simulink model "rectifysinglephase"  (Simulink 7.8)
settings: Solver=ode45  StartTime=0.0  StopTime=0.1  RelTol=1e-3
libraries: powerlib x9
settings Model: Creator=Administrator  LastModifiedBy=赵
settings DebuggingCC: FcnCallInpInsideContextMsg=Use local settings  StrictBusMsg=Warning

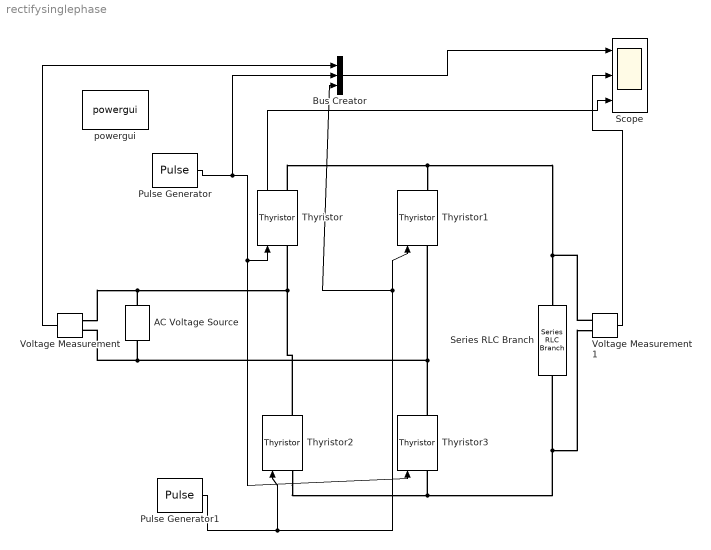
== system rectifysinglephase ==
  AC Voltage Source : powerlib/Electrical Sources/AC Voltage Source  Amplitude=100  Phase=0  Frequency=50  SampleTime=0  Measurements=None
  Bus Creator : BusCreator  Inputs=3
  Pulse Generator : DiscretePulseGenerator  PulseType=Time based  Amplitude=10  Period=0.02  PulseWidth=10  PhaseDelay=60/360*0.02
  Pulse Generator1 : DiscretePulseGenerator  PulseType=Time based  Amplitude=10  Period=0.02  PulseWidth=10  PhaseDelay=(60+180)/360*0.02
  Scope : Scope  NumInputPorts=3
      settings: YMin=-5~-5~-5  YMax=5~5~5
  Series RLC Branch : powerlib/Elements/Series RLC Branch  LConnTagsString=__new0  RConnTagsString=__new0  BranchType=RL  Resistance=2  Inductance=1  SetiL0=off  InitialCurrent=0  Capacitance=1e-6  Setx0=off  InitialVoltage=0  Measurements=None
  Thyristor{,1..3} (4 alike) : powerlib/Power Electronics/Thyristor  Ron=0.001  Lon=0  Vf=0.8  IC=0  Rs=500  Cs=250e-9  Measurements=on
  Voltage Measurement : powerlib/Measurements/Voltage Measurement  PhasorSimulation=off  OutputType=Complex  PSBequivalent=0
  Voltage Measurement1 : powerlib/Measurements/Voltage Measurement  PhasorSimulation=off  OutputType=Complex  PSBequivalent=0
  powergui : powerlib/powergui  Priority=1  SimulationMode=Continuous  SolverType=Tustin  SampleTime=50e-6  frequency=60  SPID=off  DisableSnubberDevices=off  DisableRonSwitches=off  DisableVfSwitches=off  SwTol=0  Interpol=off  DisplayEquations=off  FunctionMessages=off  frequencyindice=50  Pbase=100e6  ErrMax=1e-4  Iterations=50  UnitsV=kV  UnitsW=MW  echomessages=off  HookPort=off  EnableUseOfTLC=off  x0status=blocks  RestoreLinks=warning  ResistiveCurrentMeasurement=off  Frange=[0:2:500]  Ylog=off  Xlog=on  ShowGrid=off  save=off  variable=ZData  ZoomFFT=on  StartTime=0.0  cycles=1  DisplayStyle=1  fundamental=60  FreqAxis=off  MaxFrequency=1000  frequencyindicesteady=1  RmsSteady=1  display=off  Ts=0  methode=off
  wires:
  Pulse Generator/1 -> Thyristor/1, Thyristor3/1, Bus Creator/2
  Pulse Generator1/1 -> Thyristor2/1, Thyristor1/1, Bus Creator/3
  Voltage Measurement/1 -> Bus Creator/1
  Bus Creator/1 -> Scope/1
  Thyristor/1 -> Scope/3
  Voltage Measurement1/1 -> Scope/2
  connections:
  Voltage Measurement/LConn1 -- Thyristor2/RConn1 -- Thyristor/LConn1 -- AC Voltage Source/RConn1
  Thyristor3/RConn1 -- Thyristor1/LConn1 -- Voltage Measurement/LConn2 -- AC Voltage Source/LConn1
  Thyristor/RConn1 -- Thyristor1/RConn1 -- Voltage Measurement1/LConn1 -- Series RLC Branch/LConn1
  Thyristor2/LConn1 -- Thyristor3/LConn1 -- Series RLC Branch/RConn1 -- Voltage Measurement1/LConn2
